simulink model "A02_L2_1"  (R2016a)
settings: Solver=ode45  StartTime=0.0  StopTime=8  RelTol=1e-3
values from neighbouring files (symbols this model uses):
  C = C2    (= 0.000225)    [A03_L2_1script.m]
  C1 = 220*10^(-6)    (= 0.00022)    [A03_L2_1script.m]
  C2 = C1+(a+5)*10^(-6)    (= 0.000225)    [A03_L2_1script.m]
  L = 0.4+0.1*(a+0.5)    (= 0.45)    [A03_L2_1script.m]
  R = R1    (= 130)    [A03_L2_1script.m]
  R1 = 120+10*(a+1)    (= 130)    [A03_L2_1script.m]
  R2 = 430-15*(a+2)    (= 400)    [A03_L2_1script.m]
libraries: simulink x4
settings Model: Creator=User  LastModifiedBy=Ana
settings DataIOCC: LimitDataPoints=on  SaveFormat=Array
settings DebuggingCC: SolverPrmCheckMsg=warning
settings HardwareCC: ProdBitPerPointer=32  ProdLargestAtomicFloat=None  ProdIntDivRoundTo=Undefined  ProdEndianess=Unspecified  ProdWordSize=32  ProdHWDeviceType=32-bit Generic
settings ModelReferenceCC: PropagateSignalLabelsOutOfModel=off
settings ConfigComp: CovModelRefEnable=Off  CovSFcnEnable=off

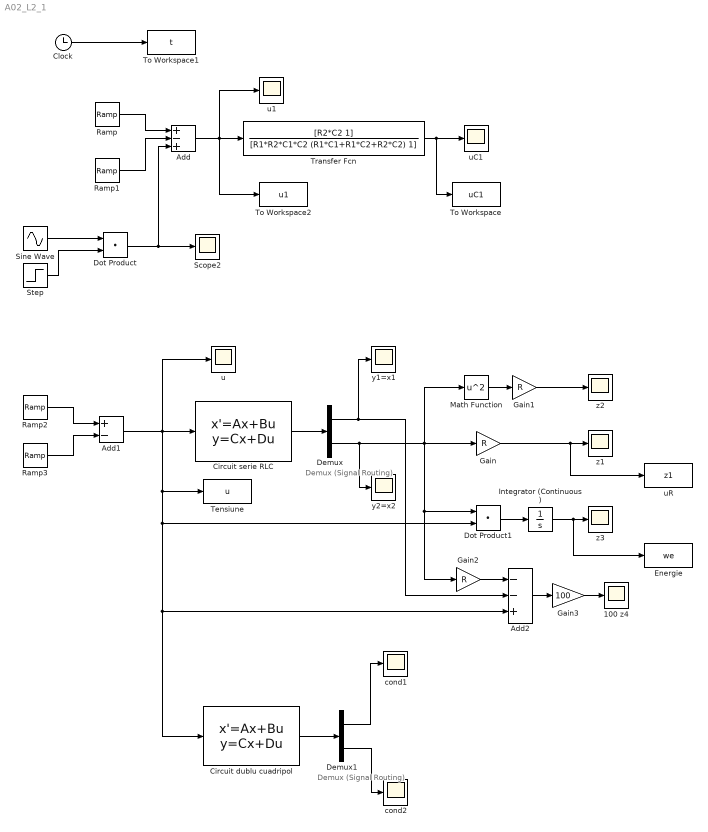
== system A02_L2_1 ==
  note: Demux
      | (Signal
      | Routing)
  note: Demux
      | (Signal
      | Routing)
  100 z4 : Scope
  Add : Sum  Inputs=+-+
  Add1 : Sum  Inputs=+-
  Add2 : Sum  Inputs=--+
  Circuit dublu cuadripol : StateSpace  A=[-(R1+R2)/(R1*R2*C1) 1/(R2*C1); 1/(R2*C2) -1/(R2*C2)]  B=[1/(R1*C1); 0]  C=[1 0; 0 1]  D=[0; 0]  X0=[0; 0]
  Circuit serie RLC : StateSpace  A=[0 1/C; -1/L -R/L]  B=[0; 1/L]  C=[1 0; 0 1]  D=[0; 0]  X0=[10; 0]
  Clock : Clock
  Demux : Demux  Outputs=2
  Demux1 : Demux  Outputs=2
  Dot Product : DotProduct  InputSameDT=on  OutDataTypeStr=Inherit: Inherit via internal rule
  Dot Product1 : DotProduct  InputSameDT=on  OutDataTypeStr=Inherit: Inherit via internal rule
  Energie : ToWorkspace  VariableName=we  SampleTime=-1
  Gain : Gain  Gain=R
  Gain1 : Gain  Gain=R
  Gain2 : Gain  Gain=R
  Gain3 : Gain  Gain=100
  Integrator (Continuous) : Integrator
  Math Function : Math  Operator=square  SaturateOnIntegerOverflow=on
  Ramp : simulink/Sources/Ramp  slope=12.5  start=1  X0=0
  Ramp1 : simulink/Sources/Ramp  slope=12.5  start=4  X0=0
  Ramp2 : simulink/Sources/Ramp  slope=12.5  start=1  X0=0
  Ramp3 : simulink/Sources/Ramp  slope=12.5  start=4  X0=0
  Scope2 : Scope
  Sine Wave : Sin  Amplitude=3  Frequency=200  SampleTime=0
  Step : Step  SampleTime=0
  Tensiune : ToWorkspace  VariableName=u  SampleTime=-1
  To Workspace : ToWorkspace  VariableName=uC1  SampleTime=-1
  To Workspace1 : ToWorkspace  VariableName=t  SampleTime=-1
  To Workspace2 : ToWorkspace  VariableName=u1  SampleTime=-1
  Transfer Fcn : TransferFcn  Numerator=[R2*C2 1]  Denominator=[R1*R2*C1*C2 (R1*C1+R1*C2+R2*C2) 1]
  cond1 : Scope
  cond2 : Scope
  u : Scope
  u1 : Scope
  uC1 : Scope
  uR : ToWorkspace  VariableName=z1  SampleTime=-1
  y1=x1 : Scope
  y2=x2 : Scope
  z1 : Scope
  z2 : Scope
  z3 : Scope
  wires:
  Transfer Fcn/1 -> To Workspace/1, uC1/1
  Clock/1 -> To Workspace1/1
  Add/1 -> To Workspace2/1, u1/1, Transfer Fcn/1
  Ramp/1 -> Add/1
  Ramp1/1 -> Add/2
  Sine Wave/1 -> Dot Product/1
  Step/1 -> Dot Product/2
  Dot Product/1 -> Scope2/1, Add/3
  Ramp2/1 -> Add1/1
  Ramp3/1 -> Add1/2
  Gain/1 -> uR/1, z1/1
  Math Function/1 -> Gain1/1
  Gain1/1 -> z2/1
  Dot Product1/1 -> Integrator (Continuous)/1
  Integrator (Continuous)/1 -> Energie/1, z3/1
  Circuit serie RLC/1 -> Demux/1
  Demux/2 -> y2=x2/1, Math Function/1, Gain2/1, Dot Product1/1, Gain/1
  Demux/1 -> y1=x1/1, Add2/2
  Gain2/1 -> Add2/1
  Add1/1 -> u/1, Tensiune/1, Circuit dublu cuadripol/1, Add2/3, Dot Product1/2, Circuit serie RLC/1
  Add2/1 -> Gain3/1
  Gain3/1 -> 100 z4/1
  Circuit dublu cuadripol/1 -> Demux1/1
  Demux1/2 -> cond2/1
  Demux1/1 -> cond1/1
